simulink model "MontajePD"  (R2021a)
settings: Solver=VariableStepAuto  StartTime=0.0  StopTime=3  MaxStep=0.05  RelTol=1e-3
libraries: pid_lib x1
settings Model: Creator=jjres  LastModifiedBy=jjres

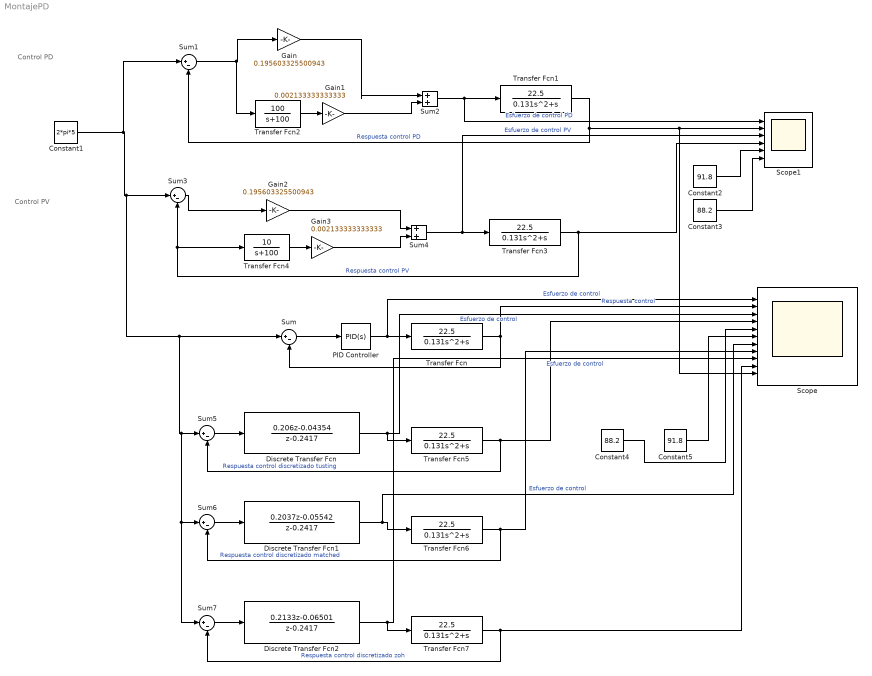
== system MontajePD ==
  note: Control PV
  note: Control PD
  Constant1 : Constant  Value=2*pi*5
  Constant2 : Constant  Value=91.8
  Constant3 : Constant  Value=88.2
  Constant4 : Constant  Value=88.2
  Constant5 : Constant  Value=91.8
  Discrete Transfer Fcn : DiscreteTransferFcn  Numerator=[0.206 -0.04354]  Denominator=[1 -0.2417]
  Discrete Transfer Fcn1 : DiscreteTransferFcn  Numerator=[0.2037 -0.05542]  Denominator=[1 -0.2417]
  Discrete Transfer Fcn2 : DiscreteTransferFcn  Numerator=[0.2133 -0.06501]  Denominator=[1 -0.2417]
  Gain : Gain  Gain=0.195603325500943
  Gain1 : Gain  Gain=0.002133333333333
  Gain2 : Gain  Gain=0.195603325500943
  Gain3 : Gain  Gain=0.002133333333333
  PID Controller : pid_lib/PID Controller  Controller=PID  Form=Parallel  TimeDomain=Continuous-time  UseExternalTs=off  SampleTime=-1  IntegratorMethod=Forward Euler  FilterMethod=Forward Euler  ControllerParametersSource=internal  P=0.195603325500943  I=0  D=0.002133333333333  UseFilter=on  N=100  TunerSelectOption=Transfer Function Based (PID Tuner App)  InitialConditionSource=internal  InitialConditionForIntegrator=0  InitialConditionForFilter=0  DifferentiatorICPrevScaledInput=0  ExternalReset=none  TrackingMode=off  Kt=1  LimitOutput=off  SatLimitsSource=internal  UpperSaturationLimit=inf  LowerSaturationLimit=-inf  LinearizeAsGain=on  AntiWindupMode=none  Kb=1  POutMin=[]  POutMax=[]  IOutMin=[]  IOutMax=[]  DOutMin=[]  DOutMax=[]  NOutMin=[]  NOutMax=[]  SumOutMin=[]  SumOutMax=[]  SaturationOutMin=[]  SaturationOutMax=[]  PParamMin=[]  PParamMax=[]  IParamMin=[]  IParamMax=[]  DParamMin=[]  DParamMax=[]  NParamMin=[]  NParamMax=[]  KbParamMin=[]  KbParamMax=[]  KtParamMin=[]  KtParamMax=[]  KbOutMin=[]  KbOutMax=[]  KtOutMin=[]  KtOutMax=[]  IntegratorOutMin=[]  IntegratorOutMax=[]  FilterOutMin=[]  FilterOutMax=[]  SumI1OutMin=[]  SumI1OutMax=[]  SumI2OutMin=[]  SumI2OutMax=[]  SumI3OutMin=[]  SumI3OutMax=[]  SumI4OutMin=[]  SumI4OutMax=[]  SumDOutMin=[]  SumDOutMax=[]  DifferentiatorOutMin=[]  DifferentiatorOutMax=[]  FilterDiffOutCoefMin=[]  FilterDiffOutCoefMax=[]  ReciprocalOutMin=[]  ReciprocalOutMax=[]  SumDenOutMin=[]  SumDenOutMax=[]  SumNumOutMin=[]  SumNumOutMax=[]  DivideOutMin=[]  DivideOutMax=[]  UdiffTsProdOutMin=[]  UdiffTsProdOutMax=[]  NTsProdOutMin=[]  NTsProdOutMax=[]  UintegralTsProdOutMin=[]  UintegralTsProdOutMax=[]  UngainTsProdOutMin=[]  UngainTsProdOutMax=[]  IntegratorContinuousStateAttributes=''  IntegratorStateMustResolveToSignalObject=off  IntegratorRTWStateStorageClass=Auto  FilterContinuousStateAttributes=''  FilterStateMustResolveToSignalObject=off  FilterRTWStateStorageClass=Auto  ParallelPVariant=InternalParameters  IdealPVariant=Disabled  IVariant=InternalParameters  DVariant=InternalParameters  IntegratorVariant=Continuous  SatVariant=Disabled  AWVariant=Passthrough  PCopyVariant=Disabled  TRVariant=Disabled  FdbkBlocksVariant=Forward  IdealPFdbkVariant=Disabled  SatFdbkVariant=Disabled  DerivativeFilterVariant=ContFilter  NVariant=InternalParameters  NCopyVariant=Disabled  FilterICVariant=InternalICsFilter  IntegratorICVariant=InternalICs  ExternalResetVariant=Disabled  TRSumVariant=Passthrough  SumFdbkVariant=Disabled  SumVariant=Sum_PID  TsampFilterVariant=InternalTs  TsampNgainVariant=Passthrough  TsampIntegralVariant=Passthrough  ExternalSaturationOutDataTypeStr=Inherit: Same as second input
  Scope : Scope  NumInputPorts=11
  Scope1 : Scope  NumInputPorts=6
  Sum{,1,3,5..7} (6 alike) : Sum  Inputs=|+-
  Sum2 : Sum  Inputs=|++
  Sum4 : Sum  Inputs=|++
  Transfer Fcn{,1,3,5..7} (6 alike) : TransferFcn  Numerator=[22.5]  Denominator=[0.131 1 0]
  Transfer Fcn2 : TransferFcn  Numerator=[100]  Denominator=[1 100]
  Transfer Fcn4 : TransferFcn  Numerator=[10]  Denominator=[1 100]
  wires:
  Sum/1 -> PID Controller/1
  PID Controller/1 -> Scope/1, Transfer Fcn/1  "Esfuerzo de control"
  Transfer Fcn/1 -> Sum/2, Scope/2  "Respuesta control"
  Gain1/1 -> Sum2/2
  Gain/1 -> Sum2/1
  Sum2/1 -> Scope1/1, Transfer Fcn1/1  "Esfuerzo de control PD"
  Transfer Fcn1/1 -> Sum1/2, Scope/11, Scope1/2  "Respuesta control PD"
  Sum1/1 -> Transfer Fcn2/1, Gain/1
  Transfer Fcn2/1 -> Gain1/1
  Transfer Fcn3/1 -> Scope1/4, Transfer Fcn4/1, Sum3/2  "Respuesta control PV"
  Gain3/1 -> Sum4/2
  Sum3/1 -> Gain2/1
  Transfer Fcn4/1 -> Gain3/1
  Gain2/1 -> Sum4/1
  Sum4/1 -> Scope1/3, Transfer Fcn3/1  "Esfuerzo de control PV"
  Constant2/1 -> Scope1/5
  Constant3/1 -> Scope1/6
  Transfer Fcn5/1 -> Scope/4, Sum5/2  "Respuesta control discretizado tusting"
  Discrete Transfer Fcn/1 -> Transfer Fcn5/1, Scope/3  "Esfuerzo de control"
  Sum5/1 -> Discrete Transfer Fcn/1
  Constant4/1 -> Scope/5
  Constant5/1 -> Scope/6
  Discrete Transfer Fcn1/1 -> Scope/7, Transfer Fcn6/1  "Esfuerzo de control"
  Sum6/1 -> Discrete Transfer Fcn1/1
  Transfer Fcn6/1 -> Scope/8, Sum6/2  "Respuesta control discretizado matched"
  Transfer Fcn7/1 -> Scope/10, Sum7/2  "Respuesta control discretizado zoh"
  Sum7/1 -> Discrete Transfer Fcn2/1
  Constant1/1 -> Sum1/1, Sum/1, Sum7/1, Sum6/1, Sum5/1, Sum3/1
  Discrete Transfer Fcn2/1 -> Scope/9, Transfer Fcn7/1  "Esfuerzo de control"
